simulink model "modelo_sistema"  (R2018b)
settings: Solver=FixedStepAuto  StartTime=0.0  StopTime=10.0  FixedStep=0.0001  RelTol=1e-3
values from neighbouring files (symbols this model uses):
  B = 100    [params.m]
  F = 10    [params.m]
  m = 100    [params.m]
libraries: simulink x1
settings Model: Creator=yasminnunes  LastModifiedBy=yasminnunes

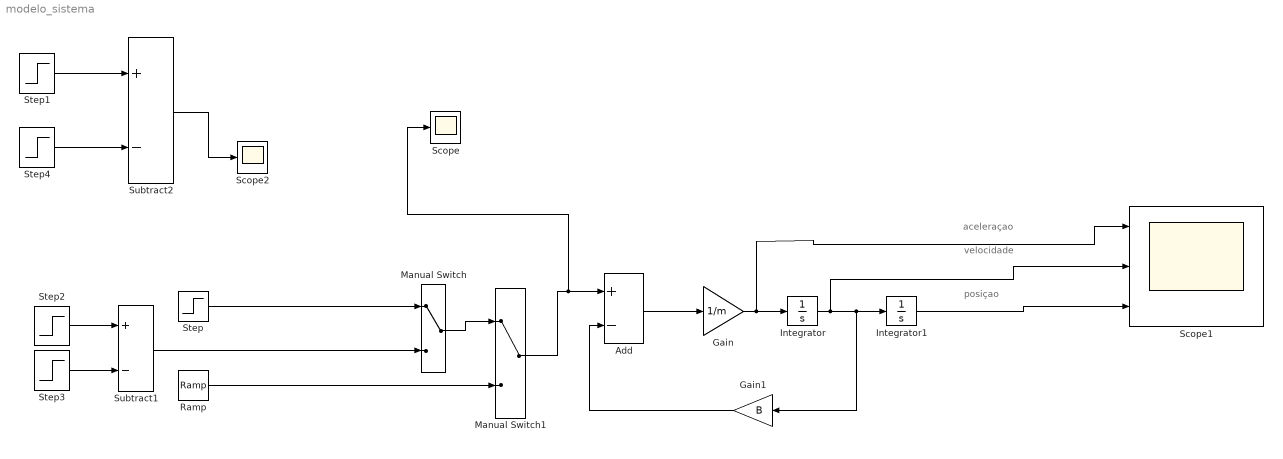
== system modelo_sistema ==
  note: aceleraçao
  note: velocidade
  note: posiçao
  Add : Sum  Inputs=+-
  Gain : Gain  Gain=1/m
  Gain1 : Gain  Gain=B
  Integrator : Integrator
  Integrator1 : Integrator
  Manual Switch : ManualSwitch
  Manual Switch1 : ManualSwitch
  Ramp : simulink/Sources/Ramp  slope=F  start=0  InitialOutput=0
  Scope : Scope
  Scope1 : Scope  NumInputPorts=3
  Scope2 : Scope
  Step : Step  After=F  SampleTime=0
  Step1 : Step  After=10  SampleTime=0
  Step2 : Step  After=F  SampleTime=0
  Step3 : Step  Time=2  After=10  SampleTime=0
  Step4 : Step  Time=1.1  After=10  SampleTime=0
  Subtract1 : Sum  Inputs=+-
  Subtract2 : Sum  Inputs=+-
  wires:
  Step/1 -> Manual Switch/1
  Add/1 -> Gain/1
  Gain/1 -> Scope1/1, Integrator/1
  Integrator/1 -> Scope1/2, Gain1/1, Integrator1/1
  Gain1/1 -> Add/2
  Integrator1/1 -> Scope1/3
  Manual Switch/1 -> Manual Switch1/1
  Ramp/1 -> Manual Switch1/2
  Manual Switch1/1 -> Scope/1, Add/1
  Subtract1/1 -> Manual Switch/2
  Step3/1 -> Subtract1/2
  Step2/1 -> Subtract1/1
  Step4/1 -> Subtract2/2
  Step1/1 -> Subtract2/1
  Subtract2/1 -> Scope2/1
